simulink model "activiry_3"  (R2024a)
settings: Solver=VariableStepAuto  StartTime=0.0  StopTime=500  RelTol=1e-3
model workspace (MAT data in the model file):
  Speed = 0
values from neighbouring files (symbols this model uses):
  cr = 0.01    [activity_3_data.m]
  g = 9.8    [activity_3_data.m]
  k_u = 4000    [activity_3_data.m]
  m = 1200    [activity_3_data.m]
  tau = 0.3    [activity_3_data.m]
settings Model: PacingRate=1000  Creator=aruns  LastModifiedBy=aruns
settings ConfigComp: CovBoundaryAbsTol=1.0e-5

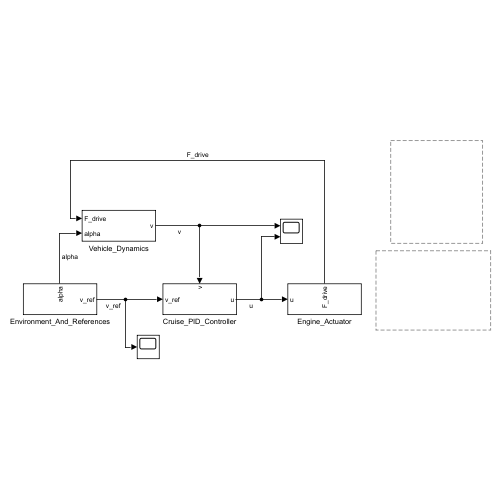
[thumbnail: Simulink's stored preview of the top-level diagram]
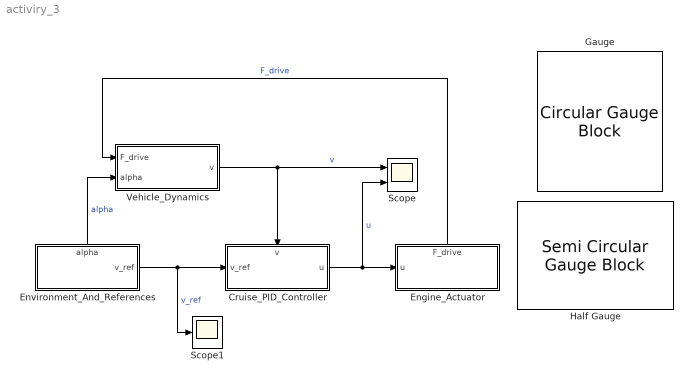
== system activiry_3 ==
  Cruise_PID_Controller : Subsystem
      settings: PortSchema="{\"entries\":[{\"content\":{\"sides\":[{\"content\":{\"connectorIds\":[\"In1\"]},\"type\":\"ConnectorPlacement.EquallySpacedRectSide\",\"uuid\":\"4f7b2cec-1f55-4aa2-adc3-78d965a4ba93\"},{\"content\":{\"connectorIds\":[\"Out1\"],\"side\":\"RIGHT\"},\"type\":\"ConnectorPlacement.EquallySpacedRectSide\",\"uuid\":\"dc063779-1c5c-4f62-b4ea-173b6becd76a\"},{\"content\":{\"connectorIds\":[\"In2\"],\"side\":\"TOP\"},\"type\":\"ConnectorPlacement.EquallySpacedRectSide\",\"uuid\":\"7c1b9744-8f2c-4f91-b29a-36cf92f7b328\"}]},\"type\":\"ConnectorPlacement.EquallySpacedConnector\",\"uuid\":\"ce9d7db3-1d7d-459b-9979-c85cf016f211\"}],\"packageUris\":[\"http://schema.mathworks.com/mf0/Connector/R2020b\"],\"version\":\"1.0\"}"
  Engine_Actuator : Subsystem
      settings: PortSchema="{\"entries\":[{\"content\":{\"sides\":[{\"content\":{\"connectorIds\":[\"In1\"]},\"type\":\"ConnectorPlacement.EquallySpacedRectSide\",\"uuid\":\"4f7b2cec-1f55-4aa2-adc3-78d965a4ba93\"},{\"content\":{\"side\":\"RIGHT\"},\"type\":\"ConnectorPlacement.EquallySpacedRectSide\",\"uuid\":\"dc063779-1c5c-4f62-b4ea-173b6becd76a\"},{\"content\":{\"connectorIds\":[\"Out1\"],\"side\":\"TOP\"},\"type\":\"ConnectorPlacement.EquallySpacedRectSide\",\"uuid\":\"7c1b9744-8f2c-4f91-b29a-36cf92f7b328\"}]},\"type\":\"ConnectorPlacement.EquallySpacedConnector\",\"uuid\":\"ce9d7db3-1d7d-459b-9979-c85cf016f211\"}],\"packageUris\":[\"http://schema.mathworks.com/mf0/Connector/R2020b\"],\"version\":\"1.0\"}"
  Environment_And_References : Subsystem
      settings: PortSchema="{\"entries\":[{\"content\":{\"sides\":[{\"content\":{},\"type\":\"ConnectorPlacement.EquallySpacedRectSide\",\"uuid\":\"ae451857-5b4e-464d-997a-c710032e5fb5\"},{\"content\":{\"connectorIds\":[\"Out1\"],\"side\":\"RIGHT\"},\"type\":\"ConnectorPlacement.EquallySpacedRectSide\",\"uuid\":\"c10e79a9-55a4-4f6b-8bb4-e981ed946527\"},{\"content\":{\"connectorIds\":[\"Out2\"],\"side\":\"TOP\"},\"type\":\"ConnectorPlacement.EquallySpacedRectSide\",\"uuid\":\"e9f7b121-8eff-44c8-a9e6-ca3a89e9c655\"}]},\"type\":\"ConnectorPlacement.EquallySpacedConnector\",\"uuid\":\"5a06232c-c315-4ccc-a6bc-b2a12fc11006\"}],\"packageUris\":[\"http://schema.mathworks.com/mf0/Connector/R2020b\"],\"version\":\"1.0\"}"
  Gauge : CircularGaugeBlock  ScaleMax=70
  Half Gauge : SemiCircularGaugeBlock  ScaleMax=1
  Scope : Scope  NumInputPorts=2
  Scope1 : Scope
  Vehicle_Dynamics : Subsystem
  wires:
  Environment_And_References/1(v_ref) -> Scope1/1, Cruise_PID_Controller/1(v_ref)  "v_ref"
  Vehicle_Dynamics/1(v) -> Scope/1, Cruise_PID_Controller/2(v)  "v"
  Cruise_PID_Controller/1(u) -> Scope/2, Engine_Actuator/1(u)  "u"
  Engine_Actuator/1(F_drive) -> Vehicle_Dynamics/1(F_drive)  "F_drive"
  Environment_And_References/2(alpha) -> Vehicle_Dynamics/2(alpha)  "alpha"

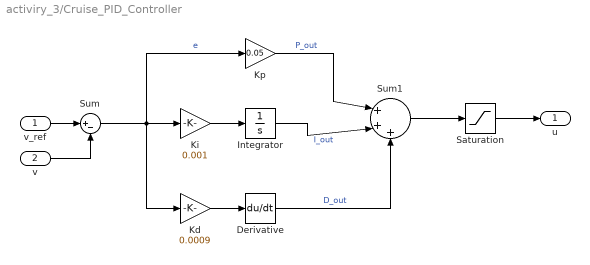
== system activiry_3/Cruise_PID_Controller ==
  v_ref : Inport
  v : Inport  Port=2
  Derivative : Derivative
  Integrator : Integrator
  Kd : Gain  Gain=0.0009
  Ki : Gain  Gain=0.001
  Kp : Gain  Gain=0.05
  Saturation : Saturate  UpperLimit=1  LowerLimit=0
  Sum : Sum  Inputs=|+-
  Sum1 : Sum  Inputs=|+++
  u : Outport
  wires:
  v_ref/1 -> Sum/1
  v/1 -> Sum/2
  Sum/1 -> Kd/1, Kp/1, Ki/1  "e"
  Ki/1 -> Integrator/1
  Kd/1 -> Derivative/1
  Kp/1 -> Sum1/1  "P_out"
  Integrator/1 -> Sum1/2  "I_out"
  Derivative/1 -> Sum1/3  "D_out"
  Sum1/1 -> Saturation/1
  Saturation/1 -> u/1

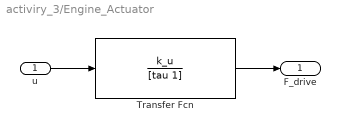
== system activiry_3/Engine_Actuator ==
  u : Inport
  Transfer Fcn : TransferFcn  Numerator=k_u  Denominator=[tau 1]
  F_drive : Outport
  wires:
  u/1 -> Transfer Fcn/1
  Transfer Fcn/1 -> F_drive/1

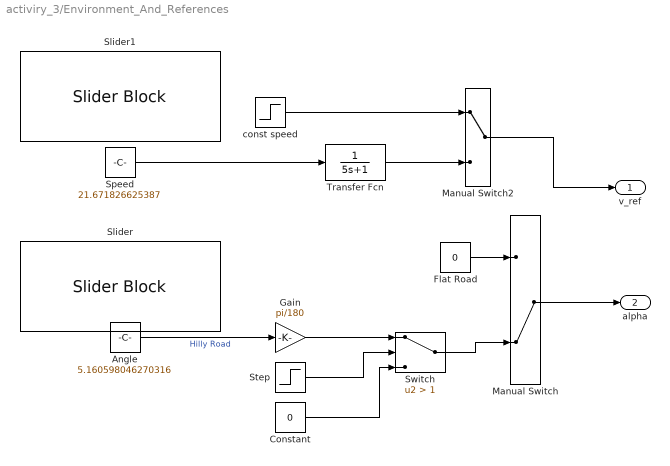
== system activiry_3/Environment_And_References ==
  Angle : Constant  Value=5.160598046270316
  Constant : Constant  Value=0
  Flat Road : Constant  Value=0
  Gain : Gain  Gain=pi/180
  Manual Switch : ManualSwitch  CurrentSetting=0
  Manual Switch2 : ManualSwitch
  Slider : SliderBlock  ScaleMin=-45  ScaleMax=45
  Slider1 : SliderBlock  ScaleMax=70
  Speed : Constant  Value=21.671826625387
  Step : Step  Time=150  After=2  SampleTime=0
  Switch : Switch  Criteria=u2 > Threshold  Threshold=1  SaturateOnIntegerOverflow=off  InputSameDT=off
  Transfer Fcn : TransferFcn  Denominator=[5 1]
  const speed : Step  Time=5  After=20  SampleTime=0
  v_ref : Outport
  alpha : Outport  Port=2
  wires:
  Flat Road/1 -> Manual Switch/1
  Manual Switch/1 -> alpha/1
  Angle/1 -> Gain/1  "Hilly Road"
  const speed/1 -> Manual Switch2/1
  Manual Switch2/1 -> v_ref/1
  Speed/1 -> Transfer Fcn/1
  Transfer Fcn/1 -> Manual Switch2/2
  Step/1 -> Switch/2
  Gain/1 -> Switch/1
  Switch/1 -> Manual Switch/2
  Constant/1 -> Switch/3

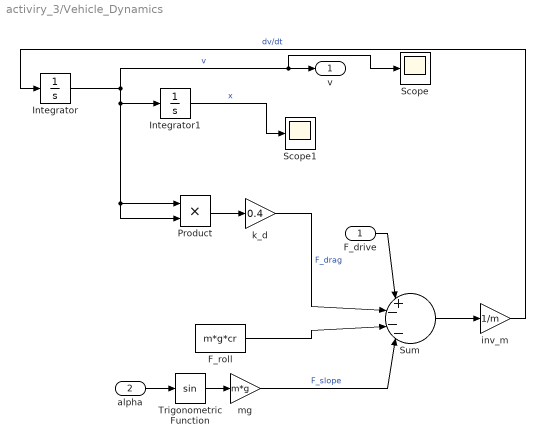
== system activiry_3/Vehicle_Dynamics ==
  F_drive : Inport
  alpha : Inport  Port=2
  F_roll : Constant  Value=m*g*cr
  Integrator : Integrator
  Integrator1 : Integrator
  Product : Product
  Scope : Scope
  Scope1 : Scope
  Sum : Sum  Inputs=|+---|
  Trigonometric Function : Trigonometry
  inv_m : Gain  Gain=1/m
  k_d : Gain  Gain=0.4
  mg : Gain  Gain=m*g
  v : Outport
  wires:
  Integrator1/1 -> Scope1/1  "x"
  Integrator/1 -> Product/2, Product/1, Integrator1/1, Scope/1, v/1  "v"
  Product/1 -> k_d/1
  k_d/1 -> Sum/2  "F_drag"
  alpha/1 -> Trigonometric Function/1
  Trigonometric Function/1 -> mg/1
  mg/1 -> Sum/4  "F_slope"
  F_drive/1 -> Sum/1
  F_roll/1 -> Sum/3
  Sum/1 -> inv_m/1
  inv_m/1 -> Integrator/1  "dv/dt"
